simulink model "DifferentialDrive"  (Simulink 8.7)
settings: Solver=VariableStepAuto  StartTime=0.0  StopTime=10.0  FixedStep=0.001  RelTol=1e-3
settings Model: Creator=maximilian  LastModifiedBy=maximilian
settings DataIOCC: LimitDataPoints=off  SaveFormat=Dataset
settings DebuggingCC: UnderspecifiedInitializationDetection=Simplified  MergeDetectMultiDrivingBlocksExec=error
settings HardwareCC: ProdBitPerPointer=64  ProdLargestAtomicFloat=Float  ProdIntDivRoundTo=Zero  ProdEndianess=LittleEndian  ProdWordSize=64  ProdHWDeviceType=Intel->x86-64 (Windows64)
settings ModelReferenceCC: PropagateSignalLabelsOutOfModel=on
settings ConfigComp: CovModelRefEnable=off

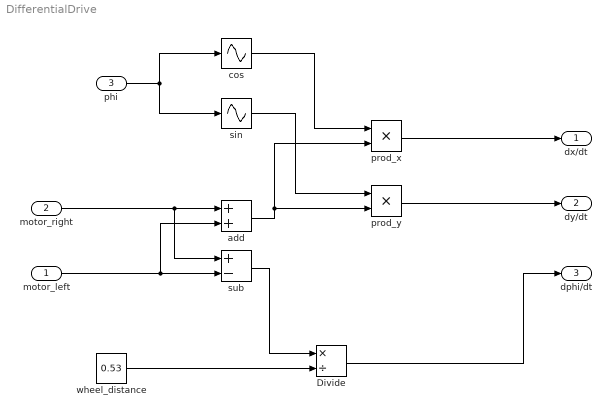
== system DifferentialDrive ==
  motor_left : Inport
  motor_right : Inport  Port=2
  phi : Inport  Port=3
  Divide : Product  Inputs=*/
  add : Sum
  cos : Sin  TimeSource=Use external signal  Amplitude=0.5  Phase=pi/2  SampleTime=0
  prod_x : Product
  prod_y : Product
  "sin " : Sin  TimeSource=Use external signal  Amplitude=0.5  SampleTime=0
  sub : Sum  Inputs=+-
  wheel_distance : Constant  Value=0.53
  dx/dt : Outport
  dy/dt : Outport  Port=2
  dphi/dt : Outport  Port=3
  wires:
  motor_left/1 -> sub/2, add/2
  motor_right/1 -> sub/1, add/1
  sub/1 -> Divide/1
  wheel_distance/1 -> Divide/2
  Divide/1 -> dphi/dt/1
  phi/1 -> "sin "/1, cos/1
  add/1 -> prod_x/2, prod_y/2
  "sin "/1 -> prod_y/1
  prod_y/1 -> dy/dt/1
  cos/1 -> prod_x/1
  prod_x/1 -> dx/dt/1
